simulink model "MotorControllers"  (R2019a)
settings: Solver=VariableStepAuto  StartTime=0.0  StopTime=10.0  RelTol=1e-3
settings Model: Creator=Dell  LastModifiedBy=Dell

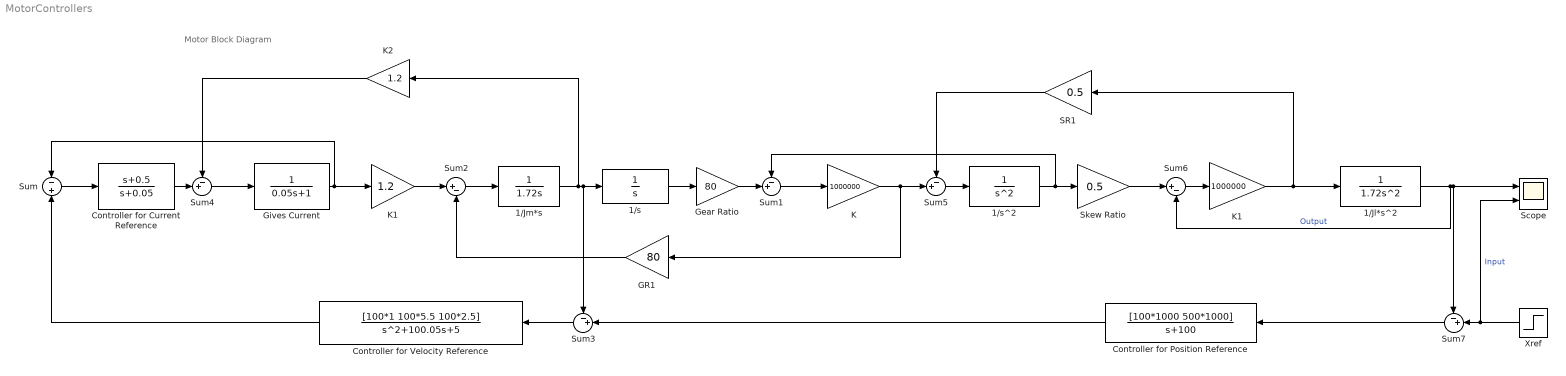
== system MotorControllers ==
  note: Motor Block Diagram
  1/Jl*s^2 : TransferFcn  Denominator=[1.72 0 0]
  1/Jm*s : TransferFcn  Denominator=[1.72 0]
  1/s : TransferFcn  Denominator=[1 0]
  1/s^2 : TransferFcn  Denominator=[1 0 0]
  Controller for Current Reference : TransferFcn  Numerator=[1 0.5]  Denominator=[1 0.05]
  Controller for Position Reference : TransferFcn  Numerator=[100*1000 500*1000]  Denominator=[1 100]
  Controller for Velocity Reference : TransferFcn  Numerator=[100*1 100*5.5 100*2.5]  Denominator=[1 100.05 5]
  GR1 : Gain  Gain=80
  Gear Ratio : Gain  Gain=80
  Gives Current : TransferFcn  Denominator=[0.05 1]
  K : Gain  Gain=1000000
  K1 : Gain  Gain=1000000
  "K1 " : Gain  Gain=1.2
  K2 : Gain  Gain=1.2
  SR1 : Gain  Gain=0.5
  Scope : Scope  NumInputPorts=2
  Skew Ratio : Gain  Gain=0.5
  Sum : Sum  Inputs=-+
  Sum{1,3..5,7} (5 alike) : Sum  Inputs=-+|
  Sum2 : Sum  Inputs=|+-
  Sum6 : Sum  Inputs=|+-
  "Xref " : Step  SampleTime=0
  wires:
  Gives Current/1 -> "K1 "/1, Sum/1
  1/Jm*s/1 -> Sum3/1, 1/s/1, K2/1
  1/s/1 -> Gear Ratio/1
  Gear Ratio/1 -> Sum1/2
  K/1 -> Sum5/2, GR1/1
  GR1/1 -> Sum2/2
  "K1 "/1 -> Sum2/1
  Sum5/1 -> 1/s^2/1
  1/s^2/1 -> Sum1/1, Skew Ratio/1
  Skew Ratio/1 -> Sum6/1
  Sum6/1 -> K1/1
  K1/1 -> SR1/1, 1/Jl*s^2/1
  1/Jl*s^2/1 -> Scope/1, Sum7/1, Sum6/2  "Output"
  SR1/1 -> Sum5/1
  Sum/1 -> Controller for Current Reference/1
  Controller for Velocity Reference/1 -> Sum/2
  Controller for Position Reference/1 -> Sum3/2
  Sum7/1 -> Controller for Position Reference/1
  "Xref "/1 -> Scope/2, Sum7/2  "Input"
  K2/1 -> Sum4/1
  Sum4/1 -> Gives Current/1
  Sum2/1 -> 1/Jm*s/1
  Sum3/1 -> Controller for Velocity Reference/1
  Controller for Current Reference/1 -> Sum4/2
  Sum1/1 -> K/1
